simulink model "SinglePanelModel"  (R2017a)
settings: Solver=ode15s  StartTime=0.0  StopTime=4  MaxStep=0.08  RelTol=1e-3
libraries: fl_lib x10, nesl_utility x10, elec_lib x6, simulink x3
settings Model: Creator=Sam  LastModifiedBy=Sam
settings OptimizationCC: DefaultParameterBehavior=Inlined  InlineInvariantSignals=on  EfficientFloat2IntCast=on
settings DebuggingCC: AssertControl=DisableAll
settings GRTTargetCC: UtilityFuncGeneration=Shared location  SupportNonFinite=off

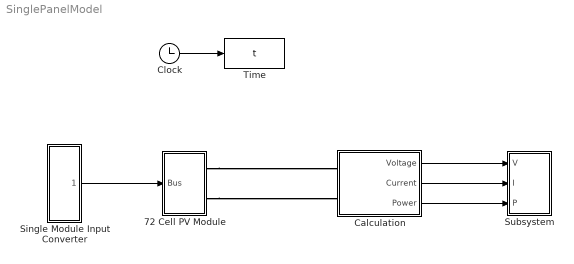
== system SinglePanelModel ==
  72 Cell PV Module : Subsystem
  Calculation : Subsystem
  Clock : Clock
      settings: Decimation=5
  Single Module Input Converter : Subsystem
  Subsystem : Subsystem
  "Time " : ToWorkspace  VariableName=t  SaveFormat=Timeseries  SampleTime=-1
  wires:
  Calculation/1(Voltage) -> Subsystem/1(V)
  Single Module Input Converter/1(Bus) -> 72 Cell PV Module/1(Bus)
  Calculation/3(Power) -> Subsystem/3(P)
  Calculation/2(Current) -> Subsystem/2(I)
  Clock/1 -> "Time "/1
  connections:
  72 Cell PV Module/RConn1 -- Calculation/LConn1
  72 Cell PV Module/RConn2 -- Calculation/LConn2

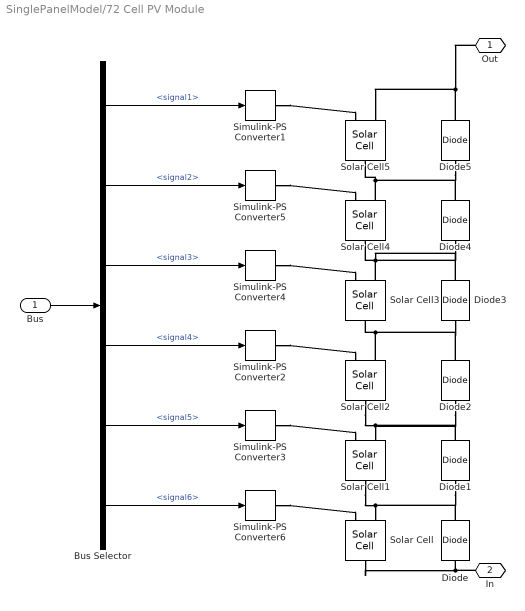
== system SinglePanelModel/72 Cell PV Module ==
  Bus : Inport
  Bus Selector : BusSelector  OutputSignals=signal1,signal2,signal3,signal4,signal5,signal6
  Diode{,1..5} (6 alike) : fl_lib/Electrical/Electrical Elements/Diode  Vf=0.6 V  Ron=0.3 Ohm  Goff=1e-8 1/Ohm  i_specify=off  i_priority=None  i=0 A  i_nominal_specify=off  i_nominal_unit=A  i_nominal_value=1  v_specify=off  v_priority=None  v=0 V  v_nominal_specify=off  v_nominal_unit=V  v_nominal_value=1
  Simulink-PS Converter{1..6} (6 alike) : nesl_utility/Simulink-PS Converter  PhysicalDomain=network_engine_domain  SubClassName=ps_input  LeftPortType=input  RightPortType=output  PseudoPeriodic=off  Frequencies=[]  NoiseDistribution=none  NoiseParameters=[]  Unit=1  AffineConversion=off  FilteringAndDerivatives=provide  SimscapeFilterOrder=1  InputFilterTimeConstant=0.001  UdotUserProvided=0
  Solar Cell{,1..5} (6 alike) : elec_lib/Sources/Solar Cell  prm=1  Isc=7.34 A  Voc=0.6 V  Is=1e-6 A  Is2=0 A  Iph=7.34 A  Ir0=1000 W/m^2  ec=1.5  N2=2  Rs=0 Ohm  Rp=Inf Ohm  N_series=12  TIPH1=0 1/K  EG=1.11 eV  TXIS1=3  TXIS2=3  TRS1=0  TRP1=0  Tmeas=25 degC  TFIXED=25 degC  thermal_mass=100 J/K  initial_temperature=25 degC
      settings: SourceProductName=Simscape Electronics  SourceProductBaseCode=SN
  Out : PMIOPort  Port=1  Side=Right
  In : PMIOPort  Port=2  Side=Right
  wires:
  Bus/1 -> Bus Selector/1
  Bus Selector/1 -> Simulink-PS Converter1/1  "<signal1>"
  Bus Selector/2 -> Simulink-PS Converter5/1  "<signal2>"
  Bus Selector/3 -> Simulink-PS Converter4/1  "<signal3>"
  Bus Selector/4 -> Simulink-PS Converter2/1  "<signal4>"
  Bus Selector/5 -> Simulink-PS Converter3/1  "<signal5>"
  Bus Selector/6 -> Simulink-PS Converter6/1  "<signal6>"
  connections:
  Simulink-PS Converter1/RConn1 -- Solar Cell5/LConn1
  Diode5/RConn1 -- Out/RConn1 -- Solar Cell5/LConn2
  Solar Cell3/LConn2 -- Diode3/RConn1 -- Diode4/LConn1 -- Solar Cell4/RConn1
  In/RConn1 -- Diode/LConn1 -- Solar Cell/RConn1
  Solar Cell1/RConn1 -- Diode1/LConn1 -- Diode/RConn1 -- Solar Cell/LConn2
  Solar Cell2/RConn1 -- Diode2/LConn1 -- Diode1/RConn1 -- Solar Cell1/LConn2
  Solar Cell2/LConn2 -- Diode2/RConn1 -- Diode3/LConn1 -- Solar Cell3/RConn1
  Solar Cell4/LConn2 -- Diode5/LConn1 -- Diode4/RConn1 -- Solar Cell5/RConn1
  Simulink-PS Converter3/RConn1 -- Solar Cell1/LConn1
  Simulink-PS Converter6/RConn1 -- Solar Cell/LConn1
  Simulink-PS Converter2/RConn1 -- Solar Cell2/LConn1
  Simulink-PS Converter4/RConn1 -- Solar Cell3/LConn1
  Simulink-PS Converter5/RConn1 -- Solar Cell4/LConn1

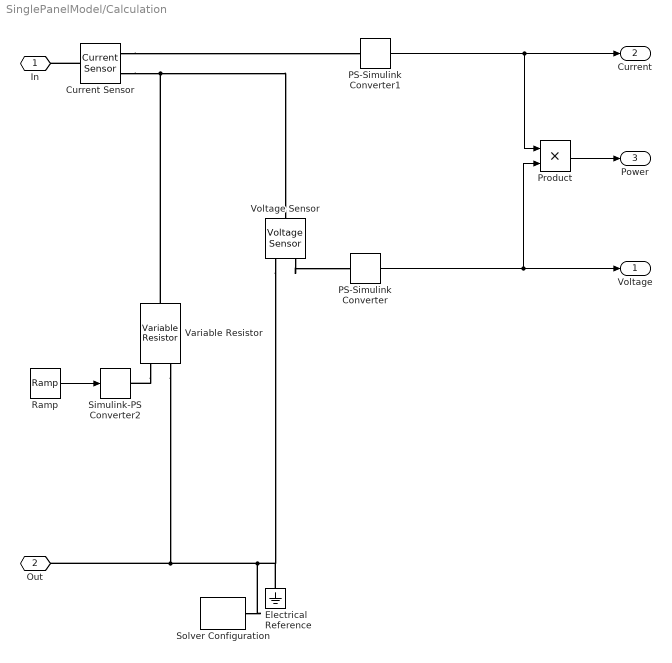
== system SinglePanelModel/Calculation ==
  Current Sensor : fl_lib/Electrical/Electrical Sensors/Current Sensor
  Electrical Reference : fl_lib/Electrical/Electrical Elements/Electrical Reference
  PS-Simulink Converter : nesl_utility/PS-Simulink Converter  PhysicalDomain=network_engine_domain  SubClassName=ps_output  LeftPortType=input  RightPortType=output  PseudoPeriodic=off  Frequencies=[]  Unit=1  AffineConversion=off
  PS-Simulink Converter1 : nesl_utility/PS-Simulink Converter  PhysicalDomain=network_engine_domain  SubClassName=ps_output  LeftPortType=input  RightPortType=output  PseudoPeriodic=off  Frequencies=[]  Unit=1  AffineConversion=off
  Product : Product
  Ramp : simulink/Sources/Ramp  slope=30  start=0  X0=0
  Simulink-PS Converter2 : nesl_utility/Simulink-PS Converter  PhysicalDomain=network_engine_domain  SubClassName=ps_input  LeftPortType=input  RightPortType=output  PseudoPeriodic=off  Frequencies=[]  NoiseDistribution=none  NoiseParameters=[]  Unit=1  AffineConversion=off  FilteringAndDerivatives=provide  SimscapeFilterOrder=1  InputFilterTimeConstant=0.001  UdotUserProvided=0
  Solver Configuration : nesl_utility/Solver Configuration  PhysicalDomain=network_engine_domain  SubClassName=solver  LeftPortType=input  RightPortType=generic  Accelerate=off  Tones=[]  Harmonics=[]  SimulateNoise=off  Profile=off  UseLocalSampling=off  EnableSwitchedLinearOptims=on  FrequencyDomain=off  UseCCode=off  RelTol=0.001  AbsTol=1e-06  MinStep=1e-09  ToWorkspace=off  RevertToSquareIcSolve=off  NumHomotopyIterations=100  PhasorMode=off  PhasorModeNumHarmonics=1  OverrideAbsTol=off  DoDC=off  ResidualTolerance=1e-09  UseLocalSolver=off  LocalSolverChoice=NE_BACKWARD_EULER_ADVANCER  LocalSolverSampleTime=0.001  DoFixedCost=off  MaxNonlinIter=3  MaxModeIter=2  LinearAlgebra=Sparse  DelaysMemoryBudget=1024  AutomaticFiltering=on  FilteringTimeConstant=0.001
  Variable Resistor : fl_lib/Electrical/Electrical Elements/Variable Resistor  Rmin=0 Ohm  i_specify=off  i_priority=None  i=0 A  i_nominal_specify=off  i_nominal_unit=A  i_nominal_value=1  v_specify=off  v_priority=None  v=0 V  v_nominal_specify=off  v_nominal_unit=V  v_nominal_value=1
  Voltage Sensor : fl_lib/Electrical/Electrical Sensors/Voltage Sensor
  In : PMIOPort  Port=1  Side=Left
  Out : PMIOPort  Port=2  Side=Left
  Voltage : Outport
  Current : Outport  Port=2
  Power : Outport  Port=3
  wires:
  Ramp/1 -> Simulink-PS Converter2/1
  PS-Simulink Converter1/1 -> Product/1, Current/1
  PS-Simulink Converter/1 -> Voltage/1, Product/2
  Product/1 -> Power/1
  connections:
  Current Sensor/LConn1 -- In/RConn1
  Current Sensor/RConn2 -- Variable Resistor/RConn1 -- Voltage Sensor/LConn1
  Solver Configuration/RConn1 -- Voltage Sensor/RConn2 -- Electrical Reference/LConn1 -- Variable Resistor/LConn2 -- Out/RConn1
  Voltage Sensor/RConn1 -- PS-Simulink Converter/LConn1
  Variable Resistor/LConn1 -- Simulink-PS Converter2/RConn1
  Current Sensor/RConn1 -- PS-Simulink Converter1/LConn1

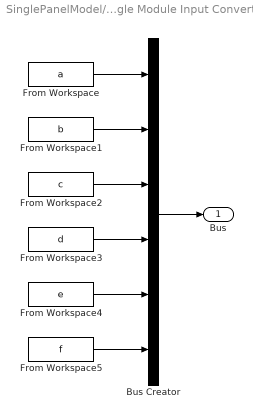
== system SinglePanelModel/Single Module Input Converter ==
  Bus Creator : BusCreator  Inputs=6
  From Workspace : FromWorkspace  VariableName=a  OutDataTypeStr=double  SampleTime=0
  From Workspace1 : FromWorkspace  VariableName=b  OutDataTypeStr=double  SampleTime=0
  From Workspace2 : FromWorkspace  VariableName=c  OutDataTypeStr=double  SampleTime=0
  From Workspace3 : FromWorkspace  VariableName=d  OutDataTypeStr=double  SampleTime=0
  From Workspace4 : FromWorkspace  VariableName=e  OutDataTypeStr=double  SampleTime=0
  From Workspace5 : FromWorkspace  VariableName=f  OutDataTypeStr=double  SampleTime=0
  Bus : Outport
  wires:
  Bus Creator/1 -> Bus/1
  From Workspace/1 -> Bus Creator/1
  From Workspace1/1 -> Bus Creator/2
  From Workspace2/1 -> Bus Creator/3
  From Workspace3/1 -> Bus Creator/4
  From Workspace4/1 -> Bus Creator/5
  From Workspace5/1 -> Bus Creator/6

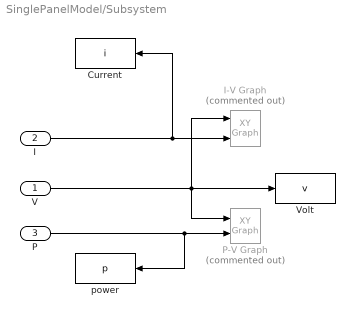
== system SinglePanelModel/Subsystem ==
  V : Inport
  I : Inport  Port=2
  P : Inport  Port=3
  Current : ToWorkspace  VariableName=i  SampleTime=-1
      settings: Save2DSignal=2-D array (concatenate along first dimension)
  "I-V Graph " : simulink/Sinks/XY Graph  Commented=on  xmin=-1  xmax=50  ymin=-1  ymax=20  st=-1
  P-V Graph : simulink/Sinks/XY Graph  Commented=on  xmin=-1  xmax=70  ymin=-1  ymax=300  st=-1
  Volt : ToWorkspace  VariableName=v  SampleTime=-1
      settings: Save2DSignal=2-D array (concatenate along first dimension)
  power : ToWorkspace  VariableName=p  SampleTime=-1
      settings: Save2DSignal=2-D array (concatenate along first dimension)
  wires:
  V/1 -> Volt/1, "I-V Graph "/1, P-V Graph/1
  I/1 -> "I-V Graph "/2, Current/1
  P/1 -> P-V Graph/2, power/1
